simulink model "sim1"  (R2024a)
settings: Solver=FixedStepAuto  StartTime=0.0  StopTime=20.0  FixedStep=1e-3  RelTol=1e-3
InitFcn:
  | k0=16;
  | k1=8;
  | a0=5;
  | a1=1;
  | b0=9;
  | b1=3;
  | theta=[k0-a0;k1-a1;b0;b1];
  | A0=[-k1 1; -k0 0];
  | A=[-a1 1; -a0 0];
  | b=[b1;b0];
  | C=[1 0];
  | D=[0;0];
settings Model: Creator=alexe  LastModifiedBy=alexe

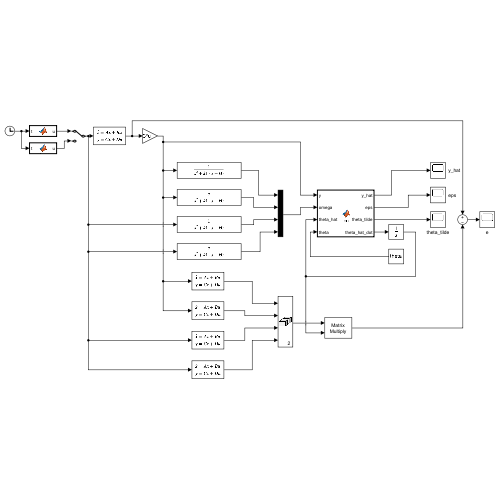
[thumbnail: Simulink's stored preview of the top-level diagram]
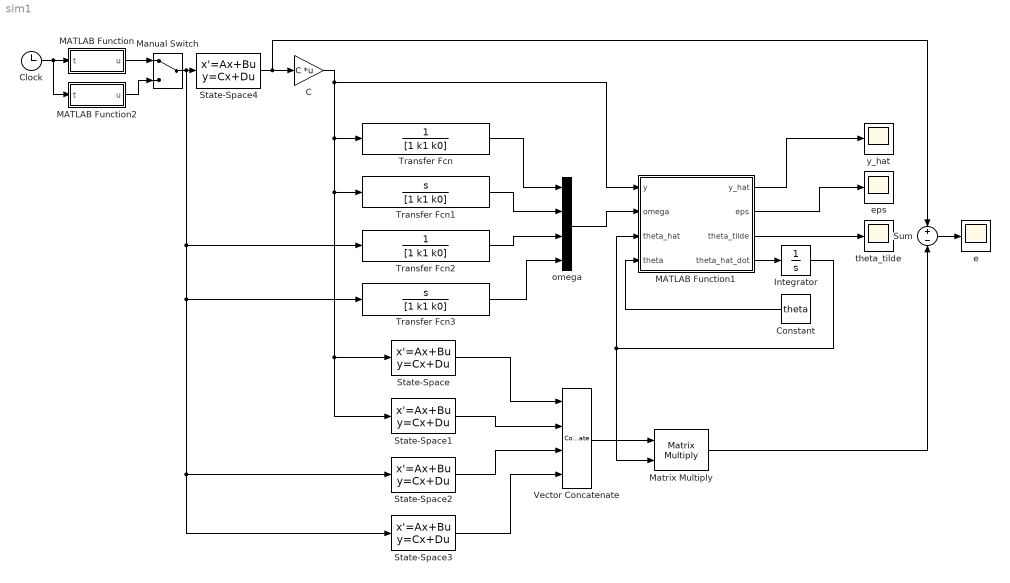
== system sim1 ==
  C : Gain  Gain=C  Multiplication=Matrix(K*u)
  Clock : Clock
  Constant : Constant  Value=theta  VectorParams1D=off
  Integrator : Integrator  InitialCondition=[0;0;0;0]
  MATLAB Function : MATLAB Function  TreatAsAtomicUnit=on
  MATLAB Function1 : MATLAB Function  TreatAsAtomicUnit=on
  MATLAB Function2 : MATLAB Function  TreatAsAtomicUnit=on
  Manual Switch : ManualSwitch
  Matrix Multiply : Product  Multiplication=Matrix(*)
  State-Space : StateSpace  A=A0  B=[0;1]  C=eye(2)  D=[0;0]  InitialCondition=[0;0];
  State-Space1 : StateSpace  A=A0  B=[1;0]  C=eye(2)  D=[0;0]  InitialCondition=[0;0];
  State-Space2 : StateSpace  A=A0  B=[0;1]  C=eye(2)  D=[0;0]  InitialCondition=[0;0];
  State-Space3 : StateSpace  A=A0  B=[1;0]  C=eye(2)  D=[0;0]  InitialCondition=[0;0];
  State-Space4 : StateSpace  A=A  B=b  C=eye(2)  D=D  InitialCondition=[0;0];
  Sum : Sum  Inputs=+-
  Transfer Fcn : TransferFcn  Numerator=[0 0 1]  Denominator=[1 k1 k0]
  Transfer Fcn1 : TransferFcn  Numerator=[0 1 0]  Denominator=[1 k1 k0]
  Transfer Fcn2 : TransferFcn  Numerator=[0 0 1]  Denominator=[1 k1 k0]
  Transfer Fcn3 : TransferFcn  Numerator=[0 1 0]  Denominator=[1 k1 k0]
  Vector Concatenate : Concatenate  NumInputs=4  Mode=Multidimensional array  ConcatenateDimension=2
  e : Scope
  eps : Scope
  omega : Mux
  theta_tilde : Scope
  y_hat : Scope
  wires:
  Transfer Fcn/1 -> omega/1
  Transfer Fcn1/1 -> omega/2
  Transfer Fcn2/1 -> omega/3
  Transfer Fcn3/1 -> omega/4
  Clock/1 -> MATLAB Function2/1(t), MATLAB Function/1(t)
  State-Space4/1 -> Sum/1, C/1
  omega/1 -> MATLAB Function1/2(omega)
  C/1 -> State-Space1/1, State-Space/1, Transfer Fcn1/1, Transfer Fcn/1, MATLAB Function1/1(y)
  State-Space/1 -> Vector Concatenate/1
  State-Space1/1 -> Vector Concatenate/2
  State-Space2/1 -> Vector Concatenate/3
  State-Space3/1 -> Vector Concatenate/4
  MATLAB Function1/1(y_hat) -> y_hat/1
  MATLAB Function1/3(theta_tilde) -> theta_tilde/1
  MATLAB Function1/2(eps) -> eps/1
  MATLAB Function1/4(theta_hat_dot) -> Integrator/1
  Integrator/1 -> MATLAB Function1/3(theta_hat), Matrix Multiply/2
  Vector Concatenate/1 -> Matrix Multiply/1
  Matrix Multiply/1 -> Sum/2
  Sum/1 -> e/1
  Constant/1 -> MATLAB Function1/4(theta)
  MATLAB Function/1(u) -> Manual Switch/1
  Manual Switch/1 -> State-Space3/1, State-Space2/1, Transfer Fcn3/1, Transfer Fcn2/1, State-Space4/1
  MATLAB Function2/1(u) -> Manual Switch/2

== matlab function sim1/MATLAB Function1 ==
  data: y input; y_hat output; omega input; theta_hat input; eps output; theta_tilde output; theta_hat_dot output; theta input
function [y_hat, eps, theta_tilde, theta_hat_dot] = fcn(y, omega, theta_hat, theta)
gamma=1;
y_hat = theta_hat'*omega;
eps = y-y_hat;
theta_tilde = theta-theta_hat;
theta_hat_dot = gamma*omega*eps;

== matlab function sim1/MATLAB Function ==
  data: t input; u output
function u = fcn(t)

u = 10*sin(t);

== matlab function sim1/MATLAB Function2 ==
  data: t input; u output
function u = fcn(t)

u = 10*sin(t)+5*cos(2*t)+4*cos(4*t)+3*cos(8*t);
